simulink model "Drone_sim"  (R2020a)
settings: Solver=FixedStepAuto  StartTime=0.0  StopTime=100  FixedStep=0.01  RelTol=1e-3
InitFcn:
  | Drone_Parameters;
values from neighbouring files (symbols this model uses):
  kp = 1    [Drone_Parameters.m]
  kR = 1    [Drone_Parameters.m]
  p0 = [0;0;0]    [Drone_Parameters.m]
  R0 = [cos(psi0) -sin(psi0) 0; sin(psi0) cos(psi0) 0; 0 0 1]    [Drone_Parameters.m]
libraries: dspmathops x2, simulink x1, simulink_extras x1
settings Model: Creator=vcichella  LastModifiedBy=vcichella

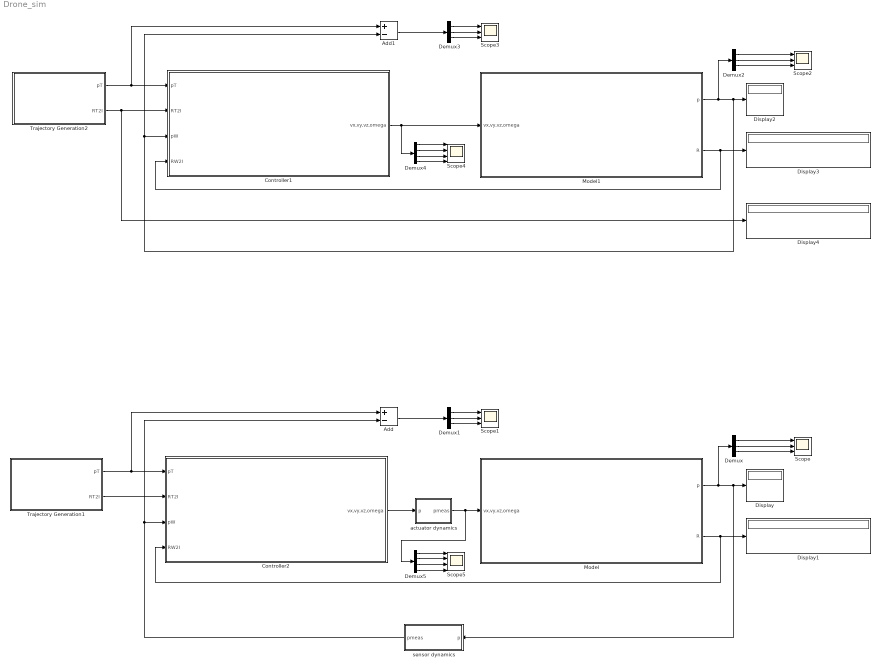
== system Drone_sim ==
  Add : Sum  Inputs=+-
  Add1 : Sum  Inputs=+-
  Controller1 : Subsystem
  Controller2 : Subsystem
  Demux{,1..3} (4 alike) : Demux  Outputs=3
  Demux4 : Demux
  Demux5 : Demux
  Display{,1..4} (5 alike) : Display
  Model : Subsystem
  Model1 : Subsystem
  Scope{,1..3} (4 alike) : Scope  NumInputPorts=3
  Scope4 : Scope  NumInputPorts=4
  Scope5 : Scope  NumInputPorts=4
  Trajectory Generation1 : Subsystem
  Trajectory Generation2 : Subsystem
  actuator dynamics : Subsystem
  sensor dynamics : Subsystem
  wires:
  Model/2(R) -> Controller2/4(RW2I), Display1/1
  Demux/1 -> Scope/1
  Demux/2 -> Scope/2
  Demux/3 -> Scope/3
  Trajectory Generation1/1("pT ") -> Controller2/1(pT), Add/1
  Trajectory Generation1/2(RT2I) -> Controller2/2(RT2I)
  Add/1 -> Demux1/1
  Demux1/1 -> Scope1/1
  Demux1/2 -> Scope1/2
  Demux1/3 -> Scope1/3
  Controller2/1(vx,vy,vz,omega) -> actuator dynamics/1(p)
  Model/1(p) -> sensor dynamics/1(p), Display/1, Demux/1
  sensor dynamics/1(pmeas) -> Controller2/3(pW), Add/2
  Model1/1(p) -> Demux2/1, Controller1/3(pW), Add1/2, Display2/1
  Controller1/1(vx,vy,vz,omega) -> Demux4/1, Model1/1(vx,vy,vz,omega)
  Demux3/3 -> Scope3/3
  Demux3/2 -> Scope3/2
  Demux3/1 -> Scope3/1
  Add1/1 -> Demux3/1
  Trajectory Generation2/1("pT ") -> Controller1/1(pT), Add1/1
  Demux2/3 -> Scope2/3
  Demux2/2 -> Scope2/2
  Demux2/1 -> Scope2/1
  Model1/2(R) -> Display3/1, Controller1/4(RW2I)
  Demux4/3 -> Scope4/3
  Demux4/2 -> Scope4/2
  Demux4/1 -> Scope4/1
  Demux4/4 -> Scope4/4
  actuator dynamics/1(pmeas) -> Demux5/1, Model/1(vx,vy,vz,omega)
  Demux5/4 -> Scope5/4
  Demux5/1 -> Scope5/1
  Demux5/2 -> Scope5/2
  Demux5/3 -> Scope5/3
  Trajectory Generation2/2(RT2I) -> Display4/1, Controller1/2(RT2I)

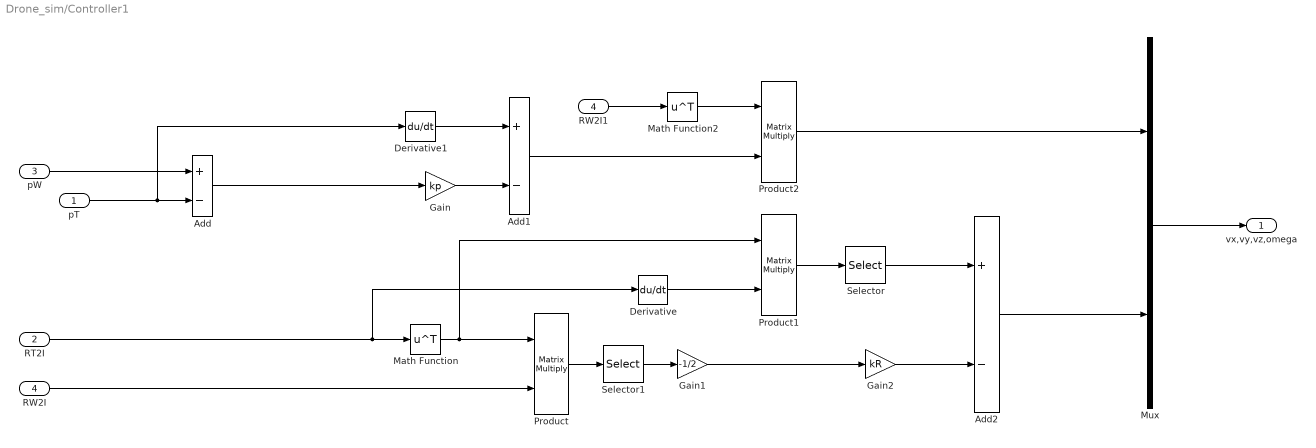
== system Drone_sim/Controller1 ==
  pT : Inport
  RT2I : Inport  Port=2
  pW : Inport  Port=3
  RW2I : Inport  Port=4
  Add : Sum  Inputs=+-
  Add1 : Sum  Inputs=+-
  Add2 : Sum  Inputs=+-
  Derivative : Derivative
  Derivative1 : Derivative
  Gain : Gain  Gain=kp
  Gain1 : Gain  Gain=-1/2
  Gain2 : Gain  Gain=kR
  Math Function : Math  Operator=transpose  SaturateOnIntegerOverflow=on
  Math Function2 : Math  Operator=transpose  SaturateOnIntegerOverflow=on
  Mux : Mux  Inputs=2
  Product : Product  Multiplication=Matrix(*)
  Product1 : Product  Multiplication=Matrix(*)
  Product2 : Product  Multiplication=Matrix(*)
  RW2I1 : InportShadow  Port=4
  Selector : Selector  NumberOfDimensions=2  InputPortWidth=9  IndexOptions=Index vector (dialog),Index vector (dialog)  Indices=2,1  OutputSizes=1,1
  Selector1 : Selector  NumberOfDimensions=2  InputPortWidth=9  IndexOptions=Index vector (dialog),Index vector (dialog)  Indices=1,2  OutputSizes=1,1
  vx,vy,vz,omega : Outport
  wires:
  Product2/1 -> Mux/1
  Gain1/1 -> Gain2/1
  Gain2/1 -> Add2/2
  Selector1/1 -> Gain1/1
  Product/1 -> Selector1/1
  Add/1 -> Gain/1
  Gain/1 -> Add1/2
  Derivative1/1 -> Add1/1
  Add1/1 -> Product2/2
  RW2I/1 -> Product/2
  Product1/1 -> Selector/1
  Derivative/1 -> Product1/2
  Math Function/1 -> Product/1, Product1/1
  RT2I/1 -> Math Function/1, Derivative/1
  pT/1 -> Add/2, Derivative1/1
  pW/1 -> Add/1
  Mux/1 -> vx,vy,vz,omega/1
  RW2I1/1 -> Math Function2/1
  Selector/1 -> Add2/1
  Add2/1 -> Mux/2
  Math Function2/1 -> Product2/1

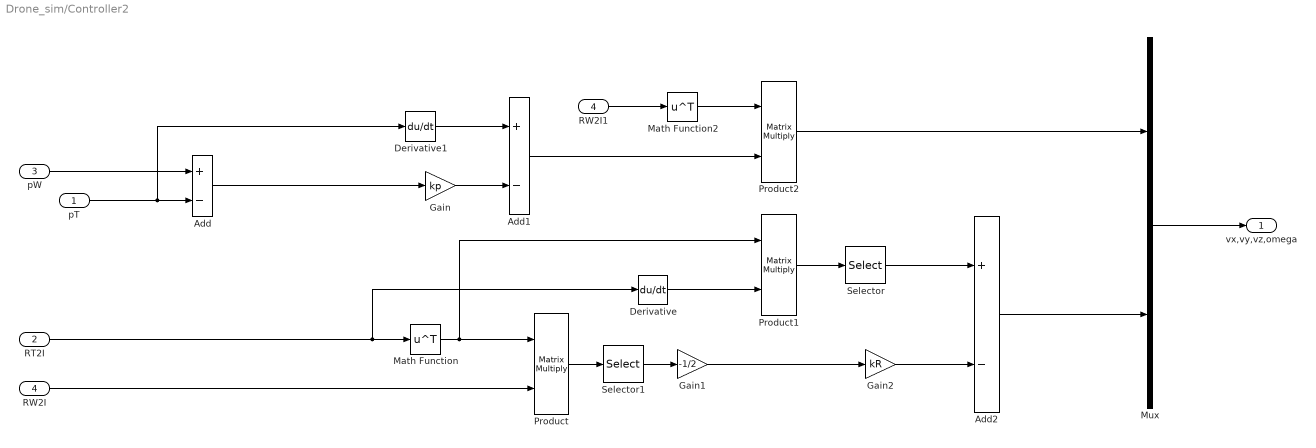
== system Drone_sim/Controller2 ==
  pT : Inport
  RT2I : Inport  Port=2
  pW : Inport  Port=3
  RW2I : Inport  Port=4
  Add : Sum  Inputs=+-
  Add1 : Sum  Inputs=+-
  Add2 : Sum  Inputs=+-
  Derivative : Derivative
  Derivative1 : Derivative
  Gain : Gain  Gain=kp
  Gain1 : Gain  Gain=-1/2
  Gain2 : Gain  Gain=kR
  Math Function : Math  Operator=transpose  SaturateOnIntegerOverflow=on
  Math Function2 : Math  Operator=transpose  SaturateOnIntegerOverflow=on
  Mux : Mux  Inputs=2
  Product : Product  Multiplication=Matrix(*)
  Product1 : Product  Multiplication=Matrix(*)
  Product2 : Product  Multiplication=Matrix(*)
  RW2I1 : InportShadow  Port=4
  Selector : Selector  NumberOfDimensions=2  InputPortWidth=9  IndexOptions=Index vector (dialog),Index vector (dialog)  Indices=2,1  OutputSizes=1,1
  Selector1 : Selector  NumberOfDimensions=2  InputPortWidth=9  IndexOptions=Index vector (dialog),Index vector (dialog)  Indices=1,2  OutputSizes=1,1
  vx,vy,vz,omega : Outport
  wires:
  Math Function2/1 -> Product2/1
  Add2/1 -> Mux/2
  Selector/1 -> Add2/1
  RW2I1/1 -> Math Function2/1
  Mux/1 -> vx,vy,vz,omega/1
  pW/1 -> Add/1
  pT/1 -> Derivative1/1, Add/2
  RT2I/1 -> Derivative/1, Math Function/1
  Math Function/1 -> Product1/1, Product/1
  Derivative/1 -> Product1/2
  Product1/1 -> Selector/1
  RW2I/1 -> Product/2
  Add1/1 -> Product2/2
  Derivative1/1 -> Add1/1
  Gain/1 -> Add1/2
  Add/1 -> Gain/1
  Product/1 -> Selector1/1
  Selector1/1 -> Gain1/1
  Gain2/1 -> Add2/2
  Gain1/1 -> Gain2/1
  Product2/1 -> Mux/1

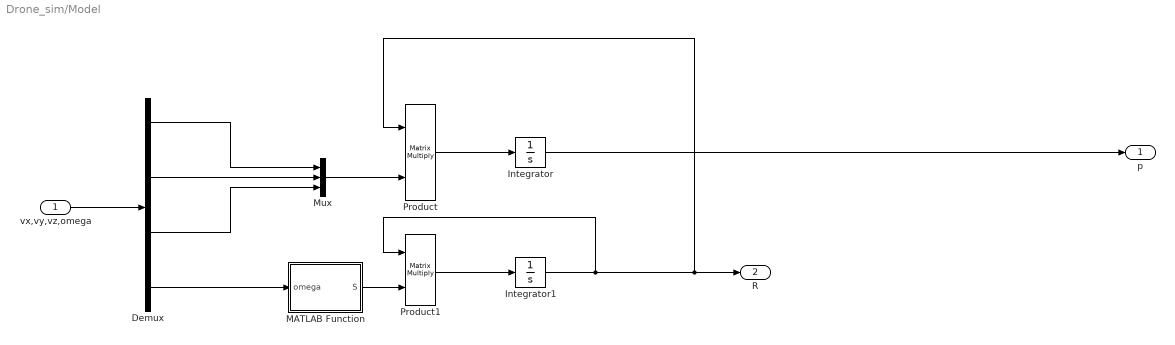
== system Drone_sim/Model ==
  vx,vy,vz,omega : Inport
  Demux : Demux
  Integrator : Integrator  InitialCondition=p0
  Integrator1 : Integrator  InitialCondition=R0
  MATLAB Function : MATLAB Function  TreatAsAtomicUnit=on
  Mux : Mux  Inputs=3
  Product : Product  Multiplication=Matrix(*)
  Product1 : Product  Multiplication=Matrix(*)
  p : Outport
  R : Outport  Port=2
  wires:
  Integrator1/1 -> Product1/1, Product/1, R/1
  vx,vy,vz,omega/1 -> Demux/1
  Product/1 -> Integrator/1
  Mux/1 -> Product/2
  Demux/1 -> Mux/1
  Demux/2 -> Mux/2
  Demux/3 -> Mux/3
  Demux/4 -> MATLAB Function/1(omega)
  Product1/1 -> Integrator1/1
  MATLAB Function/1(S) -> Product1/2
  Integrator/1 -> p/1

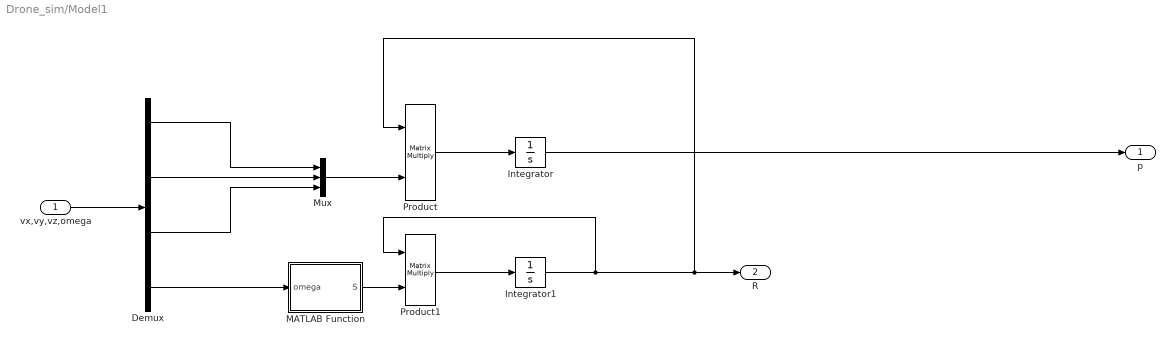
== system Drone_sim/Model1 ==
  vx,vy,vz,omega : Inport
  Demux : Demux
  Integrator : Integrator  InitialCondition=p0
  Integrator1 : Integrator  InitialCondition=R0
  MATLAB Function : MATLAB Function  TreatAsAtomicUnit=on
  Mux : Mux  Inputs=3
  Product : Product  Multiplication=Matrix(*)
  Product1 : Product  Multiplication=Matrix(*)
  p : Outport
  R : Outport  Port=2
  wires:
  Integrator/1 -> p/1
  MATLAB Function/1(S) -> Product1/2
  Product1/1 -> Integrator1/1
  Demux/4 -> MATLAB Function/1(omega)
  Demux/3 -> Mux/3
  Demux/2 -> Mux/2
  Demux/1 -> Mux/1
  Mux/1 -> Product/2
  Product/1 -> Integrator/1
  vx,vy,vz,omega/1 -> Demux/1
  Integrator1/1 -> R/1, Product/1, Product1/1

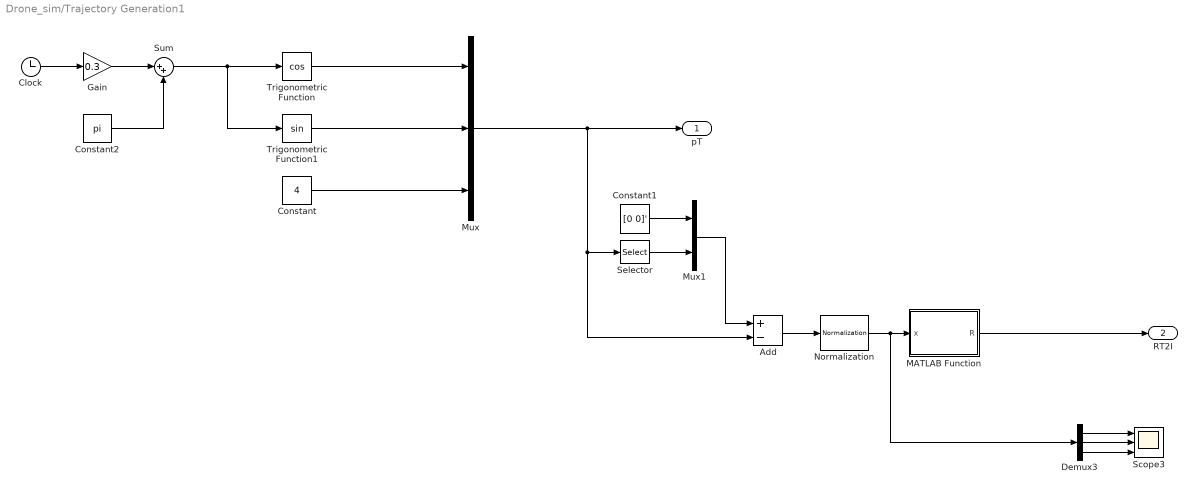
== system Drone_sim/Trajectory Generation1 ==
  Add : Sum  Inputs=+-
  Clock : Clock
  Constant : Constant  Value=4
  Constant1 : Constant  Value=[0 0]'
  Constant2 : Constant  Value=pi
  Demux3 : Demux  Outputs=3
  Gain : Gain  Gain=0.3
  MATLAB Function : MATLAB Function  TreatAsAtomicUnit=on
  Mux : Mux  Inputs=3
  Mux1 : Mux  Inputs=2
  Normalization : dspmathops/Normalization  NormType=2-norm  Bias=1e-10  NormOver=Each column  Dimension=1  roundingMode=Floor  overflowMode=off  accumDataTypeStr=Inherit: Same as product output  accumLastDataTypeStr=Inherit: Same as product output  outputDataTypeStr=Inherit: Same as product output  outputMin=[]  outputMax=[]  outputLastDataTypeStr=Inherit: Same as product output
  Scope3 : Scope  NumInputPorts=3
  Selector : Selector  InputPortWidth=3  IndexOptions=Index vector (dialog)  Indices=3  OutputSizes=1
  Sum : Sum  Inputs=|++
  Trigonometric Function : Trigonometry  Operator=cos
  Trigonometric Function1 : Trigonometry
  "pT " : Outport
  RT2I : Outport  Port=2
  wires:
  Constant2/1 -> Sum/2
  Sum/1 -> Trigonometric Function/1, Trigonometric Function1/1
  Gain/1 -> Sum/1
  Trigonometric Function/1 -> Mux/1
  Demux3/3 -> Scope3/3
  Demux3/2 -> Scope3/2
  Demux3/1 -> Scope3/1
  Mux1/1 -> Add/1
  Mux/1 -> Add/2, Selector/1, "pT "/1
  Selector/1 -> Mux1/2
  Constant1/1 -> Mux1/1
  Normalization/1 -> MATLAB Function/1(x), Demux3/1
  MATLAB Function/1(R) -> RT2I/1
  Constant/1 -> Mux/3
  Trigonometric Function1/1 -> Mux/2
  Clock/1 -> Gain/1
  Add/1 -> Normalization/1

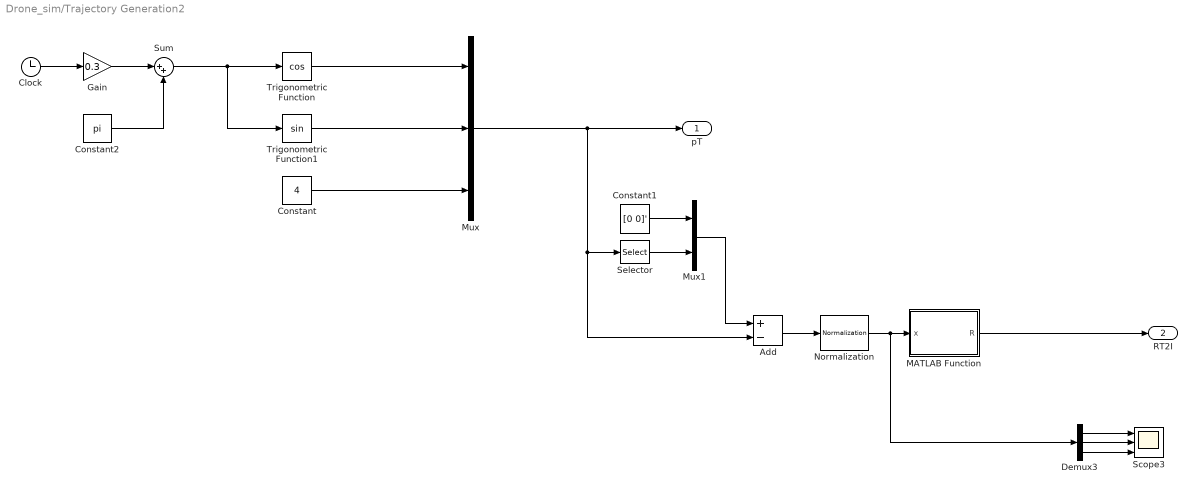
== system Drone_sim/Trajectory Generation2 ==
  Add : Sum  Inputs=+-
  Clock : Clock
  Constant : Constant  Value=4
  Constant1 : Constant  Value=[0 0]'
  Constant2 : Constant  Value=pi
  Demux3 : Demux  Outputs=3
  Gain : Gain  Gain=0.3
  MATLAB Function : MATLAB Function  TreatAsAtomicUnit=on
  Mux : Mux  Inputs=3
  Mux1 : Mux  Inputs=2
  Normalization : dspmathops/Normalization  NormType=2-norm  Bias=1e-10  NormOver=Each column  Dimension=1  roundingMode=Floor  overflowMode=off  accumDataTypeStr=Inherit: Same as product output  accumLastDataTypeStr=Inherit: Same as product output  outputDataTypeStr=Inherit: Same as product output  outputMin=[]  outputMax=[]  outputLastDataTypeStr=Inherit: Same as product output
  Scope3 : Scope  NumInputPorts=3
  Selector : Selector  InputPortWidth=3  IndexOptions=Index vector (dialog)  Indices=3  OutputSizes=1
  Sum : Sum  Inputs=|++
  Trigonometric Function : Trigonometry  Operator=cos
  Trigonometric Function1 : Trigonometry
  "pT " : Outport
  RT2I : Outport  Port=2
  wires:
  Add/1 -> Normalization/1
  Clock/1 -> Gain/1
  Trigonometric Function1/1 -> Mux/2
  Constant/1 -> Mux/3
  MATLAB Function/1(R) -> RT2I/1
  Normalization/1 -> Demux3/1, MATLAB Function/1(x)
  Constant1/1 -> Mux1/1
  Selector/1 -> Mux1/2
  Mux/1 -> "pT "/1, Selector/1, Add/2
  Mux1/1 -> Add/1
  Demux3/1 -> Scope3/1
  Demux3/2 -> Scope3/2
  Demux3/3 -> Scope3/3
  Trigonometric Function/1 -> Mux/1
  Gain/1 -> Sum/1
  Sum/1 -> Trigonometric Function1/1, Trigonometric Function/1
  Constant2/1 -> Sum/2

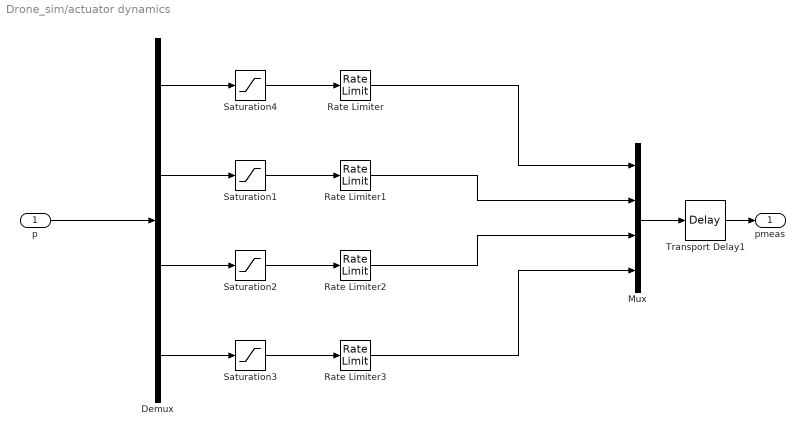
== system Drone_sim/actuator dynamics ==
  p : Inport
  Demux : Demux
  Mux : Mux
  Rate Limiter : RateLimiter  RisingSlewLimit=0.5  FallingSlewLimit=-0.5  SampleTimeMode=inherited
  Rate Limiter1 : RateLimiter  RisingSlewLimit=0.5  FallingSlewLimit=-0.5  SampleTimeMode=inherited
  Rate Limiter2 : RateLimiter  RisingSlewLimit=0.5  FallingSlewLimit=-0.5  SampleTimeMode=inherited
  Rate Limiter3 : RateLimiter  RisingSlewLimit=0.1  FallingSlewLimit=-0.1  SampleTimeMode=inherited
  Saturation1 : Saturate  UpperLimit=1  LowerLimit=-1
  Saturation2 : Saturate  UpperLimit=1  LowerLimit=-1
  Saturation3 : Saturate  UpperLimit=0.4  LowerLimit=-0.4
  Saturation4 : Saturate  UpperLimit=1  LowerLimit=-1
  Transport Delay1 : TransportDelay  DelayTime=0.1
  pmeas : Outport
  wires:
  p/1 -> Demux/1
  Transport Delay1/1 -> pmeas/1
  Mux/1 -> Transport Delay1/1
  Demux/1 -> Saturation4/1
  Demux/2 -> Saturation1/1
  Demux/3 -> Saturation2/1
  Demux/4 -> Saturation3/1
  Saturation4/1 -> Rate Limiter/1
  Saturation1/1 -> Rate Limiter1/1
  Saturation2/1 -> Rate Limiter2/1
  Saturation3/1 -> Rate Limiter3/1
  Rate Limiter1/1 -> Mux/2
  Rate Limiter2/1 -> Mux/3
  Rate Limiter/1 -> Mux/1
  Rate Limiter3/1 -> Mux/4

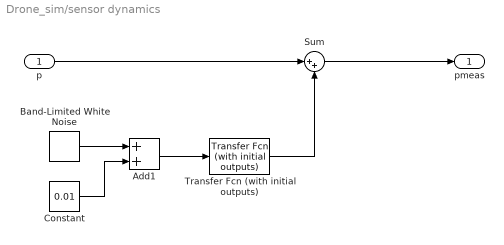
== system Drone_sim/sensor dynamics ==
  p : Inport
  Add1 : Sum
  Band-Limited White Noise : simulink/Sources/Band-Limited White Noise  Cov=[0.1]  Ts=0.1  seed=[23341]
  Constant : Constant  Value=0.01
  Sum : Sum  Inputs=|++
  Transfer Fcn (with initial outputs) : simulink_extras/Additional Linear/Transfer Fcn (with initial outputs)  N=[0.1]  D="[1  0.1]"  Y0=0.1  U0=0
  pmeas : Outport
  wires:
  Band-Limited White Noise/1 -> Add1/1
  Constant/1 -> Add1/2
  Add1/1 -> Transfer Fcn (with initial outputs)/1
  Transfer Fcn (with initial outputs)/1 -> Sum/2
  Sum/1 -> pmeas/1
  p/1 -> Sum/1

== matlab function Drone_sim/Model/MATLAB Function ==
  data: omega input; S output
function S = fcn(omega)

S = [0 -omega 0 ; omega 0 0; 0 0 0];

== matlab function Drone_sim/Trajectory Generation2/MATLAB Function ==
  data: x input; R output
function R = fcn(x)

y = [-x(2) x(1) 0]';
z = [0 0 1]';

R = [x y z];
%R = eye(3);

== matlab function Drone_sim/Trajectory Generation1/MATLAB Function ==
  data: x input; R output
function R = fcn(x)

y = [-x(2) x(1) 0]';
z = [0 0 1]';

R = [x y z];
%R = eye(3);

== matlab function Drone_sim/Model1/MATLAB Function ==
  data: omega input; S output
function S = fcn(omega)

S = [0 -omega 0 ; omega 0 0; 0 0 0];
